simulink model "poxi_model"  (R2015a)
settings: Solver=ode4  StartTime=0.0  StopTime=10  FixedStep=T  RelTol=1e-3
PreLoadFcn:
  | poxi_init
values from neighbouring files (symbols this model uses):
  T = .001    (= 0.001)    [poxi_init.m]
undefined symbols (not defined in the file or in its folder): AH, AHC, AL, ALC, BH, BHC, BL, BLC
settings Model: CovSFcnEnable=off  Creator=mueller  LastModifiedBy=Yarib
settings DebuggingCC: UnderspecifiedInitializationDetection=Classic  MergeDetectMultiDrivingBlocksExec=none  SolverPrmCheckMsg=warning

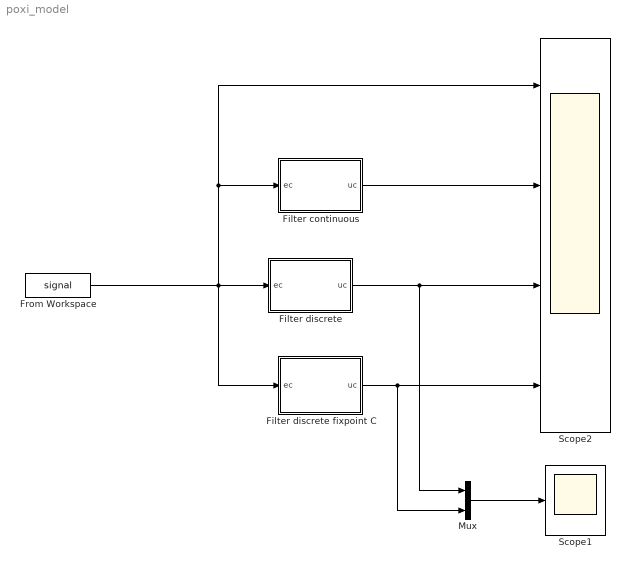
== system poxi_model ==
  Filter continuous : Subsystem
  Filter discrete : Subsystem
  Filter discrete fixpoint C : Subsystem
  From Workspace : FromWorkspace  VariableName=signal  OutDataTypeStr=double  SampleTime=T
  Mux : Mux  Inputs=2
  Scope1 : Scope
      settings: TimeRange=5  YMin=0  YMax=0.003  MaxDataPoints=10000
  Scope2 : Scope  NumInputPorts=4
      settings: TimeRange=5  YMin=0~-5~-5~-5  YMax=0.003~5~5~5  MaxDataPoints=10000
  wires:
  Filter discrete fixpoint C/1(uc) -> Scope2/4, Mux/2
  From Workspace/1 -> Filter continuous/1(ec), Scope2/1, Filter discrete fixpoint C/1(ec), Filter discrete/1(ec)
  Mux/1 -> Scope1/1
  Filter discrete/1(uc) -> Mux/1, Scope2/3
  Filter continuous/1(uc) -> Scope2/2

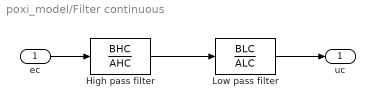
== system poxi_model/Filter continuous ==
  ec : Inport
  High pass filter : TransferFcn  Numerator=BHC  Denominator=AHC
  Low pass filter : TransferFcn  Numerator=BLC  Denominator=ALC
  uc : Outport
  wires:
  ec/1 -> High pass filter/1
  High pass filter/1 -> Low pass filter/1
  Low pass filter/1 -> uc/1

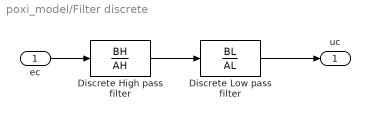
== system poxi_model/Filter discrete ==
  ec : Inport
  Discrete High pass filter : DiscreteTransferFcn  Numerator=BH  Denominator=AH  SampleTime=T
  Discrete Low pass filter : DiscreteTransferFcn  Numerator=BL  Denominator=AL  SampleTime=T
  uc : Outport
  wires:
  ec/1 -> Discrete High pass filter/1
  Discrete High pass filter/1 -> Discrete Low pass filter/1
  Discrete Low pass filter/1 -> uc/1

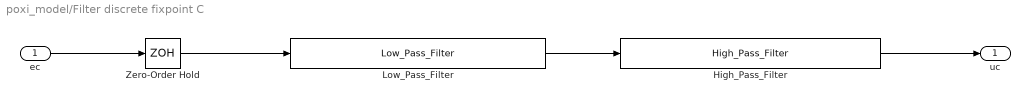
== system poxi_model/Filter discrete fixpoint C ==
  ec : Inport
  High_Pass_Filter : S-Function  FunctionName=High_Pass_Filter  mask(Legacy Function){SFunctionSpec=double y1 = high_pass_filter_wrapper(double u1), ShowSpec=on}
      mask prompts: ShowSpec "Display function specification"
      mask help:
      | This block allows you to call the legacy functions specified by the following Legacy Code Tool definition:
      | def.SFunctionName = 'High_Pass_Filter';
      | def.OutputFcnSpec = 'double y1 = high_pass_filter_wrapper(double u1)';
      | def.HeaderFiles = {'MATLAB.H', 'filter.h', 'DSP.H'};
      | def.SourceFiles = {'MATLAB.C', 'filter.c'};
      | def.IncPaths = {'..\poxi.sdk\poxi\src\dsp\'};
      | def.SrcPaths = {'..\poxi.sdk\poxi\src\dsp\'};
      mask Help: <p>This block was generated automatically by the Legacy Code Tool. For detailed help on this tool, call<a href="matlab:legacy_code('help')"> legacy_code('help')</a>.</p>
      mask Callback ShowSpec:
      | if strcmp(get_param(gcbh, 'ShowSpec'), 'on')
      |   set_param(gcbh, 'MaskDisplay', sprintf('fprintf(''%s'');', get_param(gcbh, 'SFunctionSpec')));
      | else
      |   set_param(gcbh, 'MaskDisplay', sprintf('fprintf(''%s'');', get_param(gcbh, 'FunctionName')));
      | end
      mask Display: fprintf('double y1 = high_pass_filter_wrapper(double u1)');
  Low_Pass_Filter : S-Function  FunctionName=Low_Pass_Filter  mask(Legacy Function){SFunctionSpec=double y1 = low_pass_filter_wrapper(double u1), ShowSpec=on}
      mask prompts: ShowSpec "Display function specification"
      mask help:
      | This block allows you to call the legacy functions specified by the following Legacy Code Tool definition:
      | def.SFunctionName = 'Low_Pass_Filter';
      | def.OutputFcnSpec = 'double y1 = low_pass_filter_wrapper(double u1)';
      | def.HeaderFiles = {'MATLAB.H', 'filter.h', 'dsp.h'};
      | def.SourceFiles = {'MATLAB.C', 'filter.c'};
      | def.IncPaths = {'..\poxi.sdk\poxi\src\dsp\'};
      | def.SrcPaths = {'..\poxi.sdk\poxi\src\dsp\'};
      mask Help: <p>This block was generated automatically by the Legacy Code Tool. For detailed help on this tool, call<a href="matlab:legacy_code('help')"> legacy_code('help')</a>.</p>
      mask Callback ShowSpec:
      | if strcmp(get_param(gcbh, 'ShowSpec'), 'on')
      |   set_param(gcbh, 'MaskDisplay', sprintf('fprintf(''%s'');', get_param(gcbh, 'SFunctionSpec')));
      | else
      |   set_param(gcbh, 'MaskDisplay', sprintf('fprintf(''%s'');', get_param(gcbh, 'FunctionName')));
      | end
      mask Display: fprintf('double y1 = low_pass_filter_wrapper(double u1)');
  Zero-Order Hold : ZeroOrderHold  SampleTime=T
  uc : Outport
  wires:
  ec/1 -> Zero-Order Hold/1
  Zero-Order Hold/1 -> Low_Pass_Filter/1
  High_Pass_Filter/1 -> uc/1
  Low_Pass_Filter/1 -> High_Pass_Filter/1
